simulink model "test_pkt_reord_10_1"  (Simulink 8.0)
settings: Solver=ode45  StartTime=0.0  StopTime=80000  RelTol=1e-3
libraries: xbsIndex_r4 x526, casper_library_misc x11, xps_library x1
(part 1 of 4)
settings Model: Creator=Jason Manley  LastModifiedBy=jmanley
settings DataIOCC: SignalLoggingSaveFormat=ModelDataLogs
settings OptimizationCC: InitFltsAndDblsToZero=on
settings DebuggingCC: FcnCallInpInsideContextMsg=UseLocalSettings  StrictBusMsg=Warning
settings GRTTargetCC: CombineOutputUpdateFcns=off  GRTInterface=on

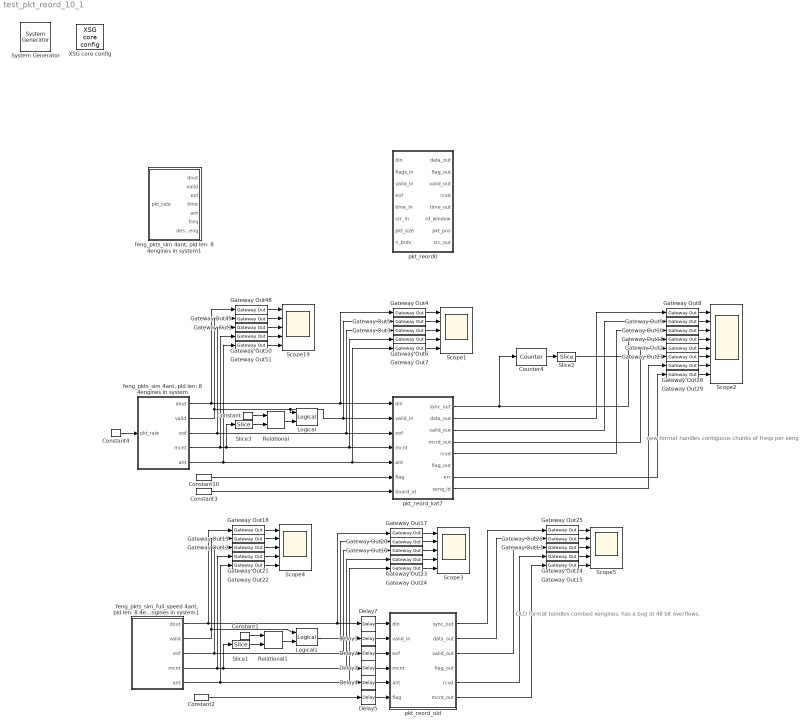
== system test_pkt_reord_10_1 ==
  note: OLD format handles combed
      | xengines. has a bug at 48 bit overflows.
  note: new format handles
      | contiguous chunks of freqs per xeng
  " System Generator" : xbsIndex_r4/ System Generator  Tag=genX  xilinxfamily=virtex2p  part=xc2vp70  speed=-7  package=ff1704  synthesis_tool=XST  clock_wrapper=Clock Enables  directory=./test_pkt_reord_10_1/sysgen  proj_type=Project Navigator  Synth_file=XST Defaults  Impl_file=ISE Defaults  testbench=off  simulink_period=1  sysclk_period=10  dcm_input_clock_period=100  incr_netlist=off  trim_vbits=Everywhere in SubSystem  dbl_ovrd=According to Block Masks  core_generation=According to Block Masks  run_coregen=off  deprecated_control=off  eval_field=0  block_type=sysgen
      settings: block_version=10.1.3
  Constant : xbsIndex_r4/Constant  const=1  gui_display_data_type=Fixed-point  arith_type=Unsigned  n_bits=2  bin_pt=0  preci_type=Single  exp_width=8  frac_width=24  explicit_period=on  period=1  equ=P=C  opselect=C  inp2=PCIN>>17  opr=+  inp1=P  carry=CIN  dbl_ovrd=off  block_type=constant
  Constant1 : xbsIndex_r4/Constant  const=0  gui_display_data_type=Fixed-point  arith_type=Unsigned  n_bits=2  bin_pt=0  preci_type=Single  exp_width=8  frac_width=24  explicit_period=off  period=1  equ=P=C  opselect=C  inp2=PCIN>>17  opr=+  inp1=P  carry=CIN  dbl_ovrd=off  block_type=constant
  Constant10 : xbsIndex_r4/Constant  const=0  gui_display_data_type=Fixed-point  arith_type=Unsigned  n_bits=1  bin_pt=0  preci_type=Single  exp_width=8  frac_width=24  explicit_period=on  period=1  equ=P=C  opselect=C  inp2=PCIN>>17  opr=+  inp1=P  carry=CIN  dbl_ovrd=off  block_type=constant
  Constant2 : xbsIndex_r4/Constant  const=0  gui_display_data_type=Fixed-point  arith_type=Unsigned  n_bits=1  bin_pt=0  preci_type=Single  exp_width=8  frac_width=24  explicit_period=on  period=1  equ=P=C  opselect=C  inp2=PCIN>>17  opr=+  inp1=P  carry=CIN  dbl_ovrd=off  block_type=constant
  Constant3 : xbsIndex_r4/Constant  const=0  gui_display_data_type=Fixed-point  arith_type=Unsigned  n_bits=32  bin_pt=0  preci_type=Single  exp_width=8  frac_width=24  explicit_period=on  period=1  equ=P=C  opselect=C  inp2=PCIN>>17  opr=+  inp1=P  carry=CIN  dbl_ovrd=off  block_type=constant
  Constant4 : xbsIndex_r4/Constant  const=1  gui_display_data_type=Fixed-point  arith_type=Unsigned  n_bits=2  bin_pt=0  preci_type=Single  exp_width=8  frac_width=24  explicit_period=off  period=1  equ=P=C  opselect=C  inp2=PCIN>>17  opr=+  inp1=P  carry=CIN  dbl_ovrd=off  block_type=constant
  Counter4 : xbsIndex_r4/Counter  cnt_type=Free Running  cnt_to=32  operation=Up  start_count=0  cnt_by_val=1  arith_type=Unsigned  n_bits=32  bin_pt=0  load_pin=off  rst=on  en=off  explicit_period=off  period=1  dbl_ovrd=off  use_behavioral_HDL=off  implementation=Fabric  use_rpm=on  block_type=counter
      settings: xl_area=[0, 0, 0, 0, 0, 0, 0]
  Delay{1..5,7} (6 alike) : xbsIndex_r4/Delay  rst=off  infoeditControl=Selection of Reset will increase slice count due to use of real FFs and instead of SRLs  en=off  latency=10  dbl_ovrd=off  reg_retiming=on  block_type=delay
      settings: xl_area=[0, 0, 0, 0, 0, 0, 0]
  Gateway Out{1..29,48..51} (33 alike) : xbsIndex_r4/Gateway Out  inherit_from_input=off  hdl_port=on  timing_constraint=None  locs_specified=off  LOCs={}  UseAsDAC=off  DACChannel='1'  block_type=gatewayout
      settings: infoedit="Gateway out block.  Converts Xilinx fixed point inputs into ouputs of type Simulink integer, double, or fixed point.<P><P>Hardware notes:  In hardware these blocks become top level output ports or are discarded, depending on how they are configured."  xl_area=[0, 0, 0, 0, 0, 0, 0]  block_version=10.1.3
  Logical : xbsIndex_r4/Logical  logical_function=AND  inputs=2  en=off  latency=0  precision=Full  arith_type=Unsigned  n_bits=16  bin_pt=0  align_bp=on  dbl_ovrd=off  block_type=logical
  Logical1 : xbsIndex_r4/Logical  logical_function=AND  inputs=2  en=off  latency=0  precision=Full  arith_type=Unsigned  n_bits=16  bin_pt=0  align_bp=on  dbl_ovrd=off  block_type=logical
  Relational : xbsIndex_r4/Relational  mode=a=b  en=off  latency=1  dbl_ovrd=off  block_type=relational
      settings: block_version=10.1.3
  Relational1 : xbsIndex_r4/Relational  mode=a=b  en=off  latency=1  dbl_ovrd=off  block_type=relational
      settings: block_version=10.1.3
  Scope{1,3..5,19} (5 alike) : Scope  NumInputPorts=5
      Scope1 settings: YMin=2e+14~0~0~0~0  YMax=1.2e+15~1~1~500~3  SaveName=ScopeData6
      Scope19 settings: YMin=0~0~0~0~0  YMax=3e+014~1~1~3000~3  SaveName=ScopeData3
      Scope3 settings: YMin=0~0~0~0~0  YMax=3e+014~1~1~3000~3  SaveName=ScopeData7
      Scope4 settings: YMin=0~0~0~0~0  YMax=3e+014~1~1~3000~3  SaveName=ScopeData8
      Scope5 settings: YMin=0~0~0~-1~-5  YMax=1~1~1~1~5  SaveName=ScopeData9
  Scope2 : Scope  NumInputPorts=8
      settings: YMin=0~0~0~-1~1~30~-1~0  YMax=4~1~1~1~7~90~1~1
  Slice1 : xbsIndex_r4/Slice  nbits=2  boolean_output=off  mode=Lower Bit Location + Width  bit1=0  base1=MSB of Input  bit0=0  base0=LSB of Input  dbl_ovrd=off  block_type=slice
      settings: infoedit="Extracts a given range of bits from each input sample and presents it at the output.  The output type is ordinarily unsigned with binary point at zero, but can be Boolean when the slice is one bit wide.<P><P>Hardware notes: In hardware this block costs nothing."  block_version=10.1.3
  Slice2 : xbsIndex_r4/Slice  nbits=32-(2+5)  boolean_output=off  mode=Lower Bit Location + Width  bit1=0  base1=MSB of Input  bit0=2+5  base0=LSB of Input  dbl_ovrd=off  block_type=slice
      settings: infoedit="Extracts a given range of bits from each input sample and presents it at the output.  The output type is ordinarily unsigned with binary point at zero, but can be Boolean when the slice is one bit wide.<P><P>Hardware notes: In hardware this block costs nothing."  block_version=10.1.3
  Slice3 : xbsIndex_r4/Slice  nbits=2  boolean_output=off  mode=Lower Bit Location + Width  bit1=8  base1=LSB of Input  bit0=6  base0=LSB of Input  dbl_ovrd=off  block_type=slice
      settings: block_version=10.1.3
  XSG core config : xps_library/XSG core config  Tag=xps:xsg  hw_sys=ROACH:sx95t  clk_src=sys_clk  ROACH_clk_src=sys_clk  ROACH2_clk_src=adc0_clk  clk_rate=100  sample_period=1  synthesis_tool=XST
  "feng_pkts_sim 4ant, pld len: 8 4engines in system" : Subsystem
  "feng_pkts_sim 4ant, pld len: 8 4engines in system1" : Subsystem
  "feng_pkts_sim_full_speed 4ant, pld len: 8 4engines in system1" : Subsystem
  pkt_reord0 : Subsystem  mask{window_bits=3, buf_bits=15}
      mask prompts: window_bits "Number of Windows to Buffer (2^?)"; buf_bits "Buffer size (2^?)"
      mask init:
      | fmtstr = sprintf('Buffer space: 2^%i words', buf_bits);
      | set_param(gcb, 'AttributesFormatString', fmtstr);
      settings: AttributesFormatString=Buffer space: 2^15 words
  pkt_reord_kat7 : Subsystem  mask{ant_bits=2, xeng_bits=3, chan_bits=8, x_int_bits=5, window_bits=3, min_sync_bits=5, share_bits=1, nx=0}
      mask prompts: ant_bits "Maximum Number of Antennas (2^?):"; xeng_bits "Number of Xengines in the system (2^?)"; chan_bits "Number of frequency channels in the system (2^?)"; x_int_bits "X Engine Integration Length (2^?):"; window_bits "Number of Windows to Buffer (2^?):"; min_sync_bits "Minimum sync period (2^n)"; share_bits "Number of Xengines on this link (2^?)"; nx "This is engine number"
      mask init:
      | sync_bits=max([min_sync_bits,chan_bits+x_int_bits+ant_bits-xeng_bits]);
      | %sync_bits=chan_bits+x_int_bits+ant_bits-xeng_bits;
      | fmtstr = sprintf('Xeng %d\nSync period: 2^%d\nPayload Len: %i', nx,sync_bits,2^(x_int_bits - 2));
      | set_param(gcb, 'AttributesFormatString', fmtstr);
      settings: AttributesFormatString=|
      | Xeng 0
      | Sync period: 2^12
      | Payload Len: 8
  pkt_reord_old : Subsystem  mask{ant_bits=2, xeng_bits=2, chan_bits=8, x_int_bits=5, window_bits=3, min_sync_bits=5}
      mask prompts: ant_bits "Maximum Number of Antennas (2^?):"; xeng_bits "Number of Xengines in the system (2^?)"; chan_bits "Number of frequency channels in the system (2^?)"; x_int_bits "X Engine Integration Length (2^?):"; window_bits "Number of Windows to Buffer (2^?):"; min_sync_bits "Minimum sync period (2^n)"
      mask init:
      | %sync_bits=max([min_sync_bits,chan_bits+x_int_bits+ant_bits-xeng_bits]);
      | sync_bits=chan_bits+x_int_bits+ant_bits-xeng_bits;
      | fmtstr = sprintf('Sync period: 2^%d\nPayload Len: %i', sync_bits,2^(x_int_bits - 2));
      | set_param(gcb, 'AttributesFormatString', fmtstr);
      settings: AttributesFormatString=|
      | Sync period: 2^13
      | Payload Len: 8
  wires:
  Gateway Out8/1 -> Scope2/1
  Gateway Out9/1 -> Scope2/2
  Gateway Out10/1 -> Scope2/3
  Gateway Out11/1 -> Scope2/4
  pkt_reord_kat7/2(data_out) -> Gateway Out8/1
  pkt_reord_kat7/3(valid_out) -> Gateway Out9/1
  pkt_reord_kat7/5(rcvd) -> Gateway Out10/1
  pkt_reord_kat7/1(sync_out) -> Gateway Out11/1, Counter4/1
  Gateway Out2/1 -> Scope2/5
  pkt_reord_kat7/4(mcnt_out) -> Gateway Out2/1
  Gateway Out48/1 -> Scope19/1
  Gateway Out49/1 -> Scope19/2
  Gateway Out50/1 -> Scope19/4
  Gateway Out51/1 -> Scope19/5
  Gateway Out1/1 -> Scope19/3
  "feng_pkts_sim 4ant, pld len: 8 4engines in system"/1(dout) -> Gateway Out48/1, Gateway Out4/1, pkt_reord_kat7/1(din)
  "feng_pkts_sim 4ant, pld len: 8 4engines in system"/2(valid) -> Gateway Out49/1, Gateway Out5/1, pkt_reord_kat7/2(valid_in), Logical/1
  "feng_pkts_sim 4ant, pld len: 8 4engines in system"/3(eof) -> Gateway Out1/1, Gateway Out3/1, pkt_reord_kat7/3(eof)
  "feng_pkts_sim 4ant, pld len: 8 4engines in system"/4(mcnt) -> Gateway Out50/1, Slice3/1, Gateway Out6/1, pkt_reord_kat7/4(mcnt)
  "feng_pkts_sim 4ant, pld len: 8 4engines in system"/5(ant) -> Gateway Out51/1, Gateway Out7/1, pkt_reord_kat7/5(ant)
  Constant10/1 -> pkt_reord_kat7/6(flag)
  Slice3/1 -> Relational/2
  Constant/1 -> Relational/1
  Relational/1 -> Logical/2
  Gateway Out4/1 -> Scope1/1
  Gateway Out5/1 -> Scope1/2
  Gateway Out6/1 -> Scope1/4
  Gateway Out7/1 -> Scope1/5
  Gateway Out3/1 -> Scope1/3
  Gateway Out25/1 -> Scope5/1
  Gateway Out26/1 -> Scope5/2
  Gateway Out13/1 -> Scope5/3
  Gateway Out14/1 -> Scope5/4
  pkt_reord_old/1(sync_out) -> Gateway Out25/1
  pkt_reord_old/2(data_out) -> Gateway Out26/1
  pkt_reord_old/5(rcvd) -> Gateway Out14/1
  Gateway Out15/1 -> Scope5/5
  pkt_reord_old/6(mcnt_out) -> Gateway Out15/1
  Gateway Out18/1 -> Scope4/1
  Gateway Out19/1 -> Scope4/2
  Gateway Out21/1 -> Scope4/4
  Gateway Out22/1 -> Scope4/5
  Gateway Out12/1 -> Scope4/3
  "feng_pkts_sim_full_speed 4ant, pld len: 8 4engines in system1"/1(dout) -> Gateway Out18/1, Gateway Out17/1, Delay7/1
  "feng_pkts_sim_full_speed 4ant, pld len: 8 4engines in system1"/2(valid) -> Gateway Out19/1, Logical1/1
  "feng_pkts_sim_full_speed 4ant, pld len: 8 4engines in system1"/3(eof) -> Gateway Out12/1, Gateway Out16/1, Delay2/1
  "feng_pkts_sim_full_speed 4ant, pld len: 8 4engines in system1"/4(mcnt) -> Gateway Out21/1, Slice1/1, Gateway Out23/1, Delay3/1
  "feng_pkts_sim_full_speed 4ant, pld len: 8 4engines in system1"/5(ant) -> Gateway Out22/1, Gateway Out24/1, Delay4/1
  Constant2/1 -> Delay5/1
  Logical1/1 -> Gateway Out20/1, Delay1/1
  Slice1/1 -> Relational1/2
  Constant1/1 -> Relational1/1
  Relational1/1 -> Logical1/2
  Gateway Out17/1 -> Scope3/1
  Gateway Out20/1 -> Scope3/2
  Gateway Out23/1 -> Scope3/4
  Gateway Out24/1 -> Scope3/5
  Gateway Out16/1 -> Scope3/3
  Delay7/1 -> pkt_reord_old/1(din)
  Delay1/1 -> pkt_reord_old/2(valid_in)
  Delay2/1 -> pkt_reord_old/3(eof)
  Delay3/1 -> pkt_reord_old/4(mcnt)
  Delay4/1 -> pkt_reord_old/5(ant)
  Delay5/1 -> pkt_reord_old/6(flag)
  pkt_reord_old/3(valid_out) -> Gateway Out13/1
  Counter4/1 -> Slice2/1
  Slice2/1 -> Gateway Out27/1
  Gateway Out27/1 -> Scope2/6
  Constant4/1 -> "feng_pkts_sim 4ant, pld len: 8 4engines in system"/1(pkt_rate)
  Constant3/1 -> pkt_reord_kat7/7(board_id)
  Gateway Out28/1 -> Scope2/7
  Gateway Out29/1 -> Scope2/8
  pkt_reord_kat7/8(xeng_id) -> Gateway Out28/1
  pkt_reord_kat7/7(err) -> Gateway Out29/1

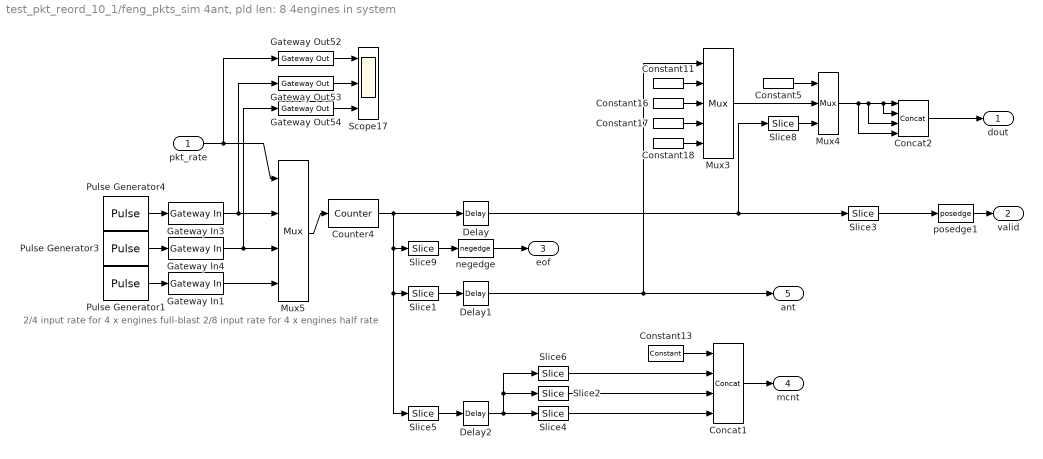
== system test_pkt_reord_10_1/feng_pkts_sim 4ant, pld len: 8 4engines in system ==
  note: 2/4 input rate for 4 x engines full-blast
      | 2/8 input rate for 4 x engines half rate
  pkt_rate : Inport
  Concat1 : xbsIndex_r4/Concat  num_inputs=4  dbl_ovrd=off  block_type=concat
      settings: block_version=10.1.3
  Concat2 : xbsIndex_r4/Concat  num_inputs=4  dbl_ovrd=off  block_type=concat
      settings: block_version=10.1.3
  Constant11 : xbsIndex_r4/Constant  const=1  gui_display_data_type=Fixed-point  arith_type=Unsigned  n_bits=16  bin_pt=0  preci_type=Single  exp_width=8  frac_width=24  explicit_period=on  period=1  equ=P=C  opselect=C  inp2=PCIN>>17  opr=+  inp1=P  carry=CIN  dbl_ovrd=off  block_type=constant
  Constant13 : xbsIndex_r4/Constant  const=0  gui_display_data_type=Fixed-point  arith_type=Unsigned  n_bits=48-(32-6)  bin_pt=0  preci_type=Single  exp_width=8  frac_width=24  explicit_period=on  period=1  equ=P=C  opselect=C  inp2=PCIN>>17  opr=+  inp1=P  carry=CIN  dbl_ovrd=off  block_type=constant
  Constant16 : xbsIndex_r4/Constant  const=2  gui_display_data_type=Fixed-point  arith_type=Unsigned  n_bits=16  bin_pt=0  preci_type=Single  exp_width=8  frac_width=24  explicit_period=on  period=1  equ=P=C  opselect=C  inp2=PCIN>>17  opr=+  inp1=P  carry=CIN  dbl_ovrd=off  block_type=constant
  Constant17 : xbsIndex_r4/Constant  const=3  gui_display_data_type=Fixed-point  arith_type=Unsigned  n_bits=16  bin_pt=0  preci_type=Single  exp_width=8  frac_width=24  explicit_period=on  period=1  equ=P=C  opselect=C  inp2=PCIN>>17  opr=+  inp1=P  carry=CIN  dbl_ovrd=off  block_type=constant
  Constant18 : xbsIndex_r4/Constant  const=4  gui_display_data_type=Fixed-point  arith_type=Unsigned  n_bits=16  bin_pt=0  preci_type=Single  exp_width=8  frac_width=24  explicit_period=on  period=1  equ=P=C  opselect=C  inp2=PCIN>>17  opr=+  inp1=P  carry=CIN  dbl_ovrd=off  block_type=constant
  Constant5 : xbsIndex_r4/Constant  const=0  gui_display_data_type=Fixed-point  arith_type=Unsigned  n_bits=1  bin_pt=0  preci_type=Single  exp_width=8  frac_width=24  explicit_period=on  period=1  equ=P=C  opselect=C  inp2=PCIN>>17  opr=+  inp1=P  carry=CIN  dbl_ovrd=off  block_type=constant
  Counter4 : xbsIndex_r4/Counter  cnt_type=Free Running  cnt_to=32  operation=Up  start_count=0  cnt_by_val=1  arith_type=Unsigned  n_bits=32  bin_pt=0  load_pin=off  rst=off  en=on  explicit_period=off  period=1  dbl_ovrd=off  use_behavioral_HDL=off  implementation=Fabric  use_rpm=on  block_type=counter
      settings: xl_area=[0, 0, 0, 0, 0, 0, 0]
  Delay : xbsIndex_r4/Delay  rst=off  infoeditControl=Selection of Reset will increase slice count due to use of real FFs and instead of SRLs  en=off  latency=1  dbl_ovrd=off  reg_retiming=off  block_type=delay
      settings: xl_area=[0, 0, 0, 0, 0, 0, 0]
  Delay1 : xbsIndex_r4/Delay  rst=off  infoeditControl=Selection of Reset will increase slice count due to use of real FFs and instead of SRLs  en=off  latency=1  dbl_ovrd=off  reg_retiming=off  block_type=delay
      settings: xl_area=[0, 0, 0, 0, 0, 0, 0]
  Delay2 : xbsIndex_r4/Delay  rst=off  infoeditControl=Selection of Reset will increase slice count due to use of real FFs and instead of SRLs  en=off  latency=1  dbl_ovrd=off  reg_retiming=off  block_type=delay
      settings: xl_area=[0, 0, 0, 0, 0, 0, 0]
  Gateway In1 : xbsIndex_r4/Gateway In  gui_display_data_type=Fixed-point  arith_type=Boolean  n_bits=8  bin_pt=6  preci_type=Single  exp_width=8  frac_width=24  quantization=Truncate  overflow=Wrap  period=1  dbl_ovrd=off  timing_constraint=None  locs_specified=off  LOCs={}  UseAsADC=off  ADCChannel='1'  inherit_from_input=off  hdl_port=on  block_type=gatewayin
      settings: infoedit="Gateway in block.  Converts inputs of type Simulink integer, double and fixed point to  Xilinx fixed point type.<P><P>Hardware notes:  In hardware these blocks become top level input ports."  xl_area=[0, 0, 0, 0, 0, 0, 0]  block_version=10.1.3
  Gateway In3 : xbsIndex_r4/Gateway In  gui_display_data_type=Fixed-point  arith_type=Boolean  n_bits=8  bin_pt=6  preci_type=Single  exp_width=8  frac_width=24  quantization=Truncate  overflow=Wrap  period=1  dbl_ovrd=off  timing_constraint=None  locs_specified=off  LOCs={}  UseAsADC=off  ADCChannel='1'  inherit_from_input=off  hdl_port=on  block_type=gatewayin
      settings: infoedit="Gateway in block.  Converts inputs of type Simulink integer, double and fixed point to  Xilinx fixed point type.<P><P>Hardware notes:  In hardware these blocks become top level input ports."  xl_area=[0, 0, 0, 0, 0, 0, 0]  block_version=10.1.3
  Gateway In4 : xbsIndex_r4/Gateway In  gui_display_data_type=Fixed-point  arith_type=Boolean  n_bits=8  bin_pt=6  preci_type=Single  exp_width=8  frac_width=24  quantization=Truncate  overflow=Wrap  period=1  dbl_ovrd=off  timing_constraint=None  locs_specified=off  LOCs={}  UseAsADC=off  ADCChannel='1'  inherit_from_input=off  hdl_port=on  block_type=gatewayin
      settings: infoedit="Gateway in block.  Converts inputs of type Simulink integer, double and fixed point to  Xilinx fixed point type.<P><P>Hardware notes:  In hardware these blocks become top level input ports."  xl_area=[0, 0, 0, 0, 0, 0, 0]  block_version=10.1.3
  Gateway Out52 : xbsIndex_r4/Gateway Out  inherit_from_input=off  hdl_port=on  timing_constraint=None  locs_specified=off  LOCs={}  UseAsDAC=off  DACChannel='1'  block_type=gatewayout
      settings: infoedit="Gateway out block.  Converts Xilinx fixed point inputs into ouputs of type Simulink integer, double, or fixed point.<P><P>Hardware notes:  In hardware these blocks become top level output ports or are discarded, depending on how they are configured."  xl_area=[0, 0, 0, 0, 0, 0, 0]  block_version=10.1.3
  Gateway Out53 : xbsIndex_r4/Gateway Out  inherit_from_input=off  hdl_port=on  timing_constraint=None  locs_specified=off  LOCs={}  UseAsDAC=off  DACChannel='1'  block_type=gatewayout
      settings: infoedit="Gateway out block.  Converts Xilinx fixed point inputs into ouputs of type Simulink integer, double, or fixed point.<P><P>Hardware notes:  In hardware these blocks become top level output ports or are discarded, depending on how they are configured."  xl_area=[0, 0, 0, 0, 0, 0, 0]  block_version=10.1.3
  Gateway Out54 : xbsIndex_r4/Gateway Out  inherit_from_input=off  hdl_port=on  timing_constraint=None  locs_specified=off  LOCs={}  UseAsDAC=off  DACChannel='1'  block_type=gatewayout
      settings: infoedit="Gateway out block.  Converts Xilinx fixed point inputs into ouputs of type Simulink integer, double, or fixed point.<P><P>Hardware notes:  In hardware these blocks become top level output ports or are discarded, depending on how they are configured."  xl_area=[0, 0, 0, 0, 0, 0, 0]  block_version=10.1.3
  Mux3 : xbsIndex_r4/Mux  inputs=4  en=off  latency=0  precision=Full  arith_type="Signed  (2's comp)"  n_bits=8  bin_pt=2  quantization=Truncate  overflow=Wrap  dbl_ovrd=off  block_type=mux
      settings: xl_area=[0, 0, 0, 0, 0, 0, 0]
  Mux4 : xbsIndex_r4/Mux  inputs=2  en=off  latency=0  precision=Full  arith_type="Signed  (2's comp)"  n_bits=8  bin_pt=2  quantization=Truncate  overflow=Wrap  dbl_ovrd=off  block_type=mux
      settings: xl_area=[0, 0, 0, 0, 0, 0, 0]
  Mux5 : xbsIndex_r4/Mux  inputs=3  en=off  latency=0  precision=Full  arith_type="Signed  (2's comp)"  n_bits=8  bin_pt=2  quantization=Truncate  overflow=Wrap  dbl_ovrd=off  block_type=mux
      settings: xl_area=[0, 0, 0, 0, 0, 0, 0]
  Pulse Generator1 : DiscretePulseGenerator  PulseWidth=2
  Pulse Generator3 : DiscretePulseGenerator  Period=4  PulseWidth=2
  Pulse Generator4 : DiscretePulseGenerator  Period=8  PulseWidth=2
  Scope17 : Scope  NumInputPorts=3
      settings: YMin=-1~0~0  YMax=1~1~1
  Slice1 : xbsIndex_r4/Slice  nbits=2  boolean_output=off  mode=Lower Bit Location + Width  bit1=0  base1=MSB of Input  bit0=4  base0=LSB of Input  dbl_ovrd=off  block_type=slice
      settings: infoedit="Extracts a given range of bits from each input sample and presents it at the output.  The output type is ordinarily unsigned with binary point at zero, but can be Boolean when the slice is one bit wide.<P><P>Hardware notes: In hardware this block costs nothing."  block_version=10.1.3
  Slice2 : xbsIndex_r4/Slice  nbits=3  boolean_output=off  mode=Lower Bit Location + Width  bit1=4+2+2  base1=LSB of Input  bit0=0  base0=LSB of Input  dbl_ovrd=off  block_type=slice
      settings: block_version=10.1.3
  Slice3 : xbsIndex_r4/Slice  nbits=1  boolean_output=on  mode=Lower Bit Location + Width  bit1=0  base1=MSB of Input  bit0=0  base0=LSB of Input  dbl_ovrd=off  block_type=slice
      settings: infoedit="Extracts a given range of bits from each input sample and presents it at the output.  The output type is ordinarily unsigned with binary point at zero, but can be Boolean when the slice is one bit wide.<P><P>Hardware notes: In hardware this block costs nothing."  block_version=10.1.3
  Slice4 : xbsIndex_r4/Slice  nbits=5  boolean_output=off  mode=Lower Bit Location + Width  bit1=0  base1=MSB of Input  bit0=3  base0=LSB of Input  dbl_ovrd=off  block_type=slice
      settings: block_version=10.1.3
  Slice5 : xbsIndex_r4/Slice  nbits=48  boolean_output=off  mode=Two Bit Locations  bit1=0  base1=MSB of Input  bit0=6  base0=LSB of Input  dbl_ovrd=off  block_type=slice
      settings: block_version=10.1.3
  Slice6 : xbsIndex_r4/Slice  nbits=10  boolean_output=off  mode=Two Bit Locations  bit1=0  base1=MSB of Input  bit0=8  base0=LSB of Input  dbl_ovrd=off  block_type=slice
      settings: block_version=10.1.3
  Slice8 : xbsIndex_r4/Slice  nbits=16  boolean_output=off  mode=Lower Bit Location + Width  bit1=0  base1=MSB of Input  bit0=1  base0=LSB of Input  dbl_ovrd=off  block_type=slice
      settings: infoedit="Extracts a given range of bits from each input sample and presents it at the output.  The output type is ordinarily unsigned with binary point at zero, but can be Boolean when the slice is one bit wide.<P><P>Hardware notes: In hardware this block costs nothing."  block_version=10.1.3
  Slice9 : xbsIndex_r4/Slice  nbits=1  boolean_output=on  mode=Lower Bit Location + Width  bit1=0  base1=MSB of Input  bit0=3  base0=LSB of Input  dbl_ovrd=off  block_type=slice
      settings: infoedit="Extracts a given range of bits from each input sample and presents it at the output.  The output type is ordinarily unsigned with binary point at zero, but can be Boolean when the slice is one bit wide.<P><P>Hardware notes: In hardware this block costs nothing."  block_version=10.1.3
  negedge : casper_library_misc/negedge  Tag=Rising Edge Detector
  posedge1 : casper_library_misc/posedge  Tag=Rising Edge Detector
  dout : Outport
  valid : Outport  Port=2
  eof : Outport  Port=3
  mcnt : Outport  Port=4
  ant : Outport  Port=5
  wires:
  Delay/1 -> Slice8/1, Slice3/1
  Concat1/1 -> mcnt/1
  posedge1/1 -> valid/1
  Concat2/1 -> dout/1
  Gateway Out54/1 -> Scope17/3
  Gateway Out53/1 -> Scope17/2
  Gateway Out52/1 -> Scope17/1
  pkt_rate/1 -> Mux5/1, Gateway Out52/1
  Gateway In4/1 -> Mux5/3, Gateway Out54/1
  Gateway In3/1 -> Mux5/2, Gateway Out53/1
  Mux5/1 -> Counter4/1
  Pulse Generator4/1 -> Gateway In3/1
  Constant5/1 -> Mux4/1
  Slice8/1 -> Mux4/3
  Mux3/1 -> Mux4/2
  Constant18/1 -> Mux3/5
  Constant17/1 -> Mux3/4
  Constant16/1 -> Mux3/3
  Constant11/1 -> Mux3/2
  Pulse Generator3/1 -> Gateway In4/1
  negedge/1 -> eof/1
  Slice9/1 -> negedge/1
  Mux4/1 -> Concat2/2, Concat2/1, Concat2/3, Concat2/4
  Counter4/1 -> Delay/1, Slice9/1, Slice1/1, Slice5/1
  Slice3/1 -> posedge1/1
  Slice1/1 -> Delay1/1
  Delay1/1 -> ant/1, Mux3/1
  Constant13/1 -> Concat1/1
  Pulse Generator1/1 -> Gateway In1/1
  Gateway In1/1 -> Mux5/4
  Delay2/1 -> Slice4/1, Slice2/1, Slice6/1
  Slice5/1 -> Delay2/1
  Slice6/1 -> Concat1/2
  Slice2/1 -> Concat1/3
  Slice4/1 -> Concat1/4

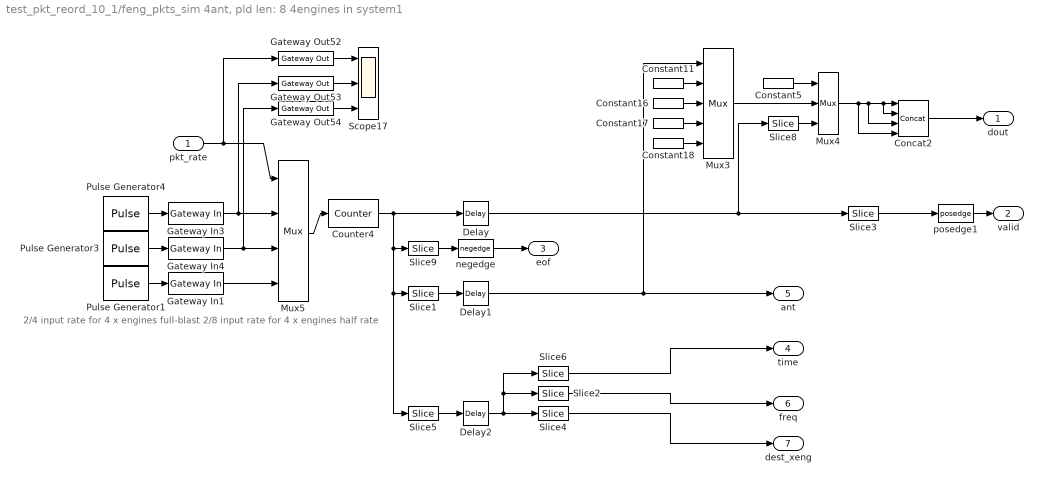
== system test_pkt_reord_10_1/feng_pkts_sim 4ant, pld len: 8 4engines in system1 ==
  note: 2/4 input rate for 4 x engines full-blast
      | 2/8 input rate for 4 x engines half rate
  pkt_rate : Inport
  Concat2 : xbsIndex_r4/Concat  num_inputs=4  dbl_ovrd=off  block_type=concat
      settings: block_version=10.1.3
  Constant11 : xbsIndex_r4/Constant  const=1  gui_display_data_type=Fixed-point  arith_type=Unsigned  n_bits=16  bin_pt=0  preci_type=Single  exp_width=8  frac_width=24  explicit_period=on  period=1  equ=P=C  opselect=C  inp2=PCIN>>17  opr=+  inp1=P  carry=CIN  dbl_ovrd=off  block_type=constant
  Constant16 : xbsIndex_r4/Constant  const=2  gui_display_data_type=Fixed-point  arith_type=Unsigned  n_bits=16  bin_pt=0  preci_type=Single  exp_width=8  frac_width=24  explicit_period=on  period=1  equ=P=C  opselect=C  inp2=PCIN>>17  opr=+  inp1=P  carry=CIN  dbl_ovrd=off  block_type=constant
  Constant17 : xbsIndex_r4/Constant  const=3  gui_display_data_type=Fixed-point  arith_type=Unsigned  n_bits=16  bin_pt=0  preci_type=Single  exp_width=8  frac_width=24  explicit_period=on  period=1  equ=P=C  opselect=C  inp2=PCIN>>17  opr=+  inp1=P  carry=CIN  dbl_ovrd=off  block_type=constant
  Constant18 : xbsIndex_r4/Constant  const=4  gui_display_data_type=Fixed-point  arith_type=Unsigned  n_bits=16  bin_pt=0  preci_type=Single  exp_width=8  frac_width=24  explicit_period=on  period=1  equ=P=C  opselect=C  inp2=PCIN>>17  opr=+  inp1=P  carry=CIN  dbl_ovrd=off  block_type=constant
  Constant5 : xbsIndex_r4/Constant  const=0  gui_display_data_type=Fixed-point  arith_type=Unsigned  n_bits=1  bin_pt=0  preci_type=Single  exp_width=8  frac_width=24  explicit_period=on  period=1  equ=P=C  opselect=C  inp2=PCIN>>17  opr=+  inp1=P  carry=CIN  dbl_ovrd=off  block_type=constant
  Counter4 : xbsIndex_r4/Counter  cnt_type=Free Running  cnt_to=32  operation=Up  start_count=0  cnt_by_val=1  arith_type=Unsigned  n_bits=32  bin_pt=0  load_pin=off  rst=off  en=on  explicit_period=off  period=1  dbl_ovrd=off  use_behavioral_HDL=off  implementation=Fabric  use_rpm=on  block_type=counter
      settings: xl_area=[0, 0, 0, 0, 0, 0, 0]
  Delay : xbsIndex_r4/Delay  rst=off  infoeditControl=Selection of Reset will increase slice count due to use of real FFs and instead of SRLs  en=off  latency=1  dbl_ovrd=off  reg_retiming=off  block_type=delay
      settings: xl_area=[0, 0, 0, 0, 0, 0, 0]
  Delay1 : xbsIndex_r4/Delay  rst=off  infoeditControl=Selection of Reset will increase slice count due to use of real FFs and instead of SRLs  en=off  latency=1  dbl_ovrd=off  reg_retiming=off  block_type=delay
      settings: xl_area=[0, 0, 0, 0, 0, 0, 0]
  Delay2 : xbsIndex_r4/Delay  rst=off  infoeditControl=Selection of Reset will increase slice count due to use of real FFs and instead of SRLs  en=off  latency=1  dbl_ovrd=off  reg_retiming=off  block_type=delay
      settings: xl_area=[0, 0, 0, 0, 0, 0, 0]
  Gateway In1 : xbsIndex_r4/Gateway In  gui_display_data_type=Fixed-point  arith_type=Boolean  n_bits=8  bin_pt=6  preci_type=Single  exp_width=8  frac_width=24  quantization=Truncate  overflow=Wrap  period=1  dbl_ovrd=off  timing_constraint=None  locs_specified=off  LOCs={}  UseAsADC=off  ADCChannel='1'  inherit_from_input=off  hdl_port=on  block_type=gatewayin
      settings: infoedit="Gateway in block.  Converts inputs of type Simulink integer, double and fixed point to  Xilinx fixed point type.<P><P>Hardware notes:  In hardware these blocks become top level input ports."  xl_area=[0, 0, 0, 0, 0, 0, 0]  block_version=10.1.3
  Gateway In3 : xbsIndex_r4/Gateway In  gui_display_data_type=Fixed-point  arith_type=Boolean  n_bits=8  bin_pt=6  preci_type=Single  exp_width=8  frac_width=24  quantization=Truncate  overflow=Wrap  period=1  dbl_ovrd=off  timing_constraint=None  locs_specified=off  LOCs={}  UseAsADC=off  ADCChannel='1'  inherit_from_input=off  hdl_port=on  block_type=gatewayin
      settings: infoedit="Gateway in block.  Converts inputs of type Simulink integer, double and fixed point to  Xilinx fixed point type.<P><P>Hardware notes:  In hardware these blocks become top level input ports."  xl_area=[0, 0, 0, 0, 0, 0, 0]  block_version=10.1.3
  Gateway In4 : xbsIndex_r4/Gateway In  gui_display_data_type=Fixed-point  arith_type=Boolean  n_bits=8  bin_pt=6  preci_type=Single  exp_width=8  frac_width=24  quantization=Truncate  overflow=Wrap  period=1  dbl_ovrd=off  timing_constraint=None  locs_specified=off  LOCs={}  UseAsADC=off  ADCChannel='1'  inherit_from_input=off  hdl_port=on  block_type=gatewayin
      settings: infoedit="Gateway in block.  Converts inputs of type Simulink integer, double and fixed point to  Xilinx fixed point type.<P><P>Hardware notes:  In hardware these blocks become top level input ports."  xl_area=[0, 0, 0, 0, 0, 0, 0]  block_version=10.1.3
  Gateway Out52 : xbsIndex_r4/Gateway Out  inherit_from_input=off  hdl_port=on  timing_constraint=None  locs_specified=off  LOCs={}  UseAsDAC=off  DACChannel='1'  block_type=gatewayout
      settings: infoedit="Gateway out block.  Converts Xilinx fixed point inputs into ouputs of type Simulink integer, double, or fixed point.<P><P>Hardware notes:  In hardware these blocks become top level output ports or are discarded, depending on how they are configured."  xl_area=[0, 0, 0, 0, 0, 0, 0]  block_version=10.1.3
  Gateway Out53 : xbsIndex_r4/Gateway Out  inherit_from_input=off  hdl_port=on  timing_constraint=None  locs_specified=off  LOCs={}  UseAsDAC=off  DACChannel='1'  block_type=gatewayout
      settings: infoedit="Gateway out block.  Converts Xilinx fixed point inputs into ouputs of type Simulink integer, double, or fixed point.<P><P>Hardware notes:  In hardware these blocks become top level output ports or are discarded, depending on how they are configured."  xl_area=[0, 0, 0, 0, 0, 0, 0]  block_version=10.1.3
  Gateway Out54 : xbsIndex_r4/Gateway Out  inherit_from_input=off  hdl_port=on  timing_constraint=None  locs_specified=off  LOCs={}  UseAsDAC=off  DACChannel='1'  block_type=gatewayout
      settings: infoedit="Gateway out block.  Converts Xilinx fixed point inputs into ouputs of type Simulink integer, double, or fixed point.<P><P>Hardware notes:  In hardware these blocks become top level output ports or are discarded, depending on how they are configured."  xl_area=[0, 0, 0, 0, 0, 0, 0]  block_version=10.1.3
  Mux3 : xbsIndex_r4/Mux  inputs=4  en=off  latency=0  precision=Full  arith_type="Signed  (2's comp)"  n_bits=8  bin_pt=2  quantization=Truncate  overflow=Wrap  dbl_ovrd=off  block_type=mux
      settings: xl_area=[0, 0, 0, 0, 0, 0, 0]
  Mux4 : xbsIndex_r4/Mux  inputs=2  en=off  latency=0  precision=Full  arith_type="Signed  (2's comp)"  n_bits=8  bin_pt=2  quantization=Truncate  overflow=Wrap  dbl_ovrd=off  block_type=mux
      settings: xl_area=[0, 0, 0, 0, 0, 0, 0]
  Mux5 : xbsIndex_r4/Mux  inputs=3  en=off  latency=0  precision=Full  arith_type="Signed  (2's comp)"  n_bits=8  bin_pt=2  quantization=Truncate  overflow=Wrap  dbl_ovrd=off  block_type=mux
      settings: xl_area=[0, 0, 0, 0, 0, 0, 0]
  Pulse Generator1 : DiscretePulseGenerator  PulseWidth=2
  Pulse Generator3 : DiscretePulseGenerator  Period=4  PulseWidth=2
  Pulse Generator4 : DiscretePulseGenerator  Period=8  PulseWidth=2
  Scope17 : Scope  NumInputPorts=3
      settings: YMin=-1~0~0  YMax=1~1~1
  Slice1 : xbsIndex_r4/Slice  nbits=2  boolean_output=off  mode=Lower Bit Location + Width  bit1=0  base1=MSB of Input  bit0=4  base0=LSB of Input  dbl_ovrd=off  block_type=slice
      settings: infoedit="Extracts a given range of bits from each input sample and presents it at the output.  The output type is ordinarily unsigned with binary point at zero, but can be Boolean when the slice is one bit wide.<P><P>Hardware notes: In hardware this block costs nothing."  block_version=10.1.3
  Slice2 : xbsIndex_r4/Slice  nbits=3  boolean_output=off  mode=Lower Bit Location + Width  bit1=4+2+2  base1=LSB of Input  bit0=0  base0=LSB of Input  dbl_ovrd=off  block_type=slice
      settings: block_version=10.1.3
  Slice3 : xbsIndex_r4/Slice  nbits=1  boolean_output=on  mode=Lower Bit Location + Width  bit1=0  base1=MSB of Input  bit0=0  base0=LSB of Input  dbl_ovrd=off  block_type=slice
      settings: infoedit="Extracts a given range of bits from each input sample and presents it at the output.  The output type is ordinarily unsigned with binary point at zero, but can be Boolean when the slice is one bit wide.<P><P>Hardware notes: In hardware this block costs nothing."  block_version=10.1.3
  Slice4 : xbsIndex_r4/Slice  nbits=5  boolean_output=off  mode=Lower Bit Location + Width  bit1=0  base1=MSB of Input  bit0=3  base0=LSB of Input  dbl_ovrd=off  block_type=slice
      settings: block_version=10.1.3
  Slice5 : xbsIndex_r4/Slice  nbits=48  boolean_output=off  mode=Two Bit Locations  bit1=0  base1=MSB of Input  bit0=6  base0=LSB of Input  dbl_ovrd=off  block_type=slice
      settings: block_version=10.1.3
  Slice6 : xbsIndex_r4/Slice  nbits=10  boolean_output=off  mode=Two Bit Locations  bit1=0  base1=MSB of Input  bit0=8  base0=LSB of Input  dbl_ovrd=off  block_type=slice
      settings: block_version=10.1.3
  Slice8 : xbsIndex_r4/Slice  nbits=16  boolean_output=off  mode=Lower Bit Location + Width  bit1=0  base1=MSB of Input  bit0=1  base0=LSB of Input  dbl_ovrd=off  block_type=slice
      settings: infoedit="Extracts a given range of bits from each input sample and presents it at the output.  The output type is ordinarily unsigned with binary point at zero, but can be Boolean when the slice is one bit wide.<P><P>Hardware notes: In hardware this block costs nothing."  block_version=10.1.3
  Slice9 : xbsIndex_r4/Slice  nbits=1  boolean_output=on  mode=Lower Bit Location + Width  bit1=0  base1=MSB of Input  bit0=3  base0=LSB of Input  dbl_ovrd=off  block_type=slice
      settings: infoedit="Extracts a given range of bits from each input sample and presents it at the output.  The output type is ordinarily unsigned with binary point at zero, but can be Boolean when the slice is one bit wide.<P><P>Hardware notes: In hardware this block costs nothing."  block_version=10.1.3
  negedge : casper_library_misc/negedge  Tag=Rising Edge Detector
  posedge1 : casper_library_misc/posedge  Tag=Rising Edge Detector
  dout : Outport
  valid : Outport  Port=2
  eof : Outport  Port=3
  time : Outport  Port=4
  ant : Outport  Port=5
  freq : Outport  Port=6
  dest_xeng : Outport  Port=7
  wires:
  Slice5/1 -> Delay2/1
  Delay2/1 -> Slice6/1, Slice2/1, Slice4/1
  Gateway In1/1 -> Mux5/4
  Pulse Generator1/1 -> Gateway In1/1
  Delay1/1 -> Mux3/1, ant/1
  Slice1/1 -> Delay1/1
  Slice3/1 -> posedge1/1
  Counter4/1 -> Slice5/1, Slice1/1, Slice9/1, Delay/1
  Mux4/1 -> Concat2/4, Concat2/3, Concat2/1, Concat2/2
  Slice9/1 -> negedge/1
  negedge/1 -> eof/1
  Pulse Generator3/1 -> Gateway In4/1
  Constant11/1 -> Mux3/2
  Constant16/1 -> Mux3/3
  Constant17/1 -> Mux3/4
  Constant18/1 -> Mux3/5
  Mux3/1 -> Mux4/2
  Slice8/1 -> Mux4/3
  Constant5/1 -> Mux4/1
  Pulse Generator4/1 -> Gateway In3/1
  Mux5/1 -> Counter4/1
  Gateway In3/1 -> Gateway Out53/1, Mux5/2
  Gateway In4/1 -> Gateway Out54/1, Mux5/3
  pkt_rate/1 -> Gateway Out52/1, Mux5/1
  Gateway Out52/1 -> Scope17/1
  Gateway Out53/1 -> Scope17/2
  Gateway Out54/1 -> Scope17/3
  Concat2/1 -> dout/1
  posedge1/1 -> valid/1
  Delay/1 -> Slice3/1, Slice8/1
  Slice2/1 -> freq/1
  Slice6/1 -> time/1
  Slice4/1 -> dest_xeng/1

== system test_pkt_reord_10_1/feng_pkts_sim_full_speed 4ant, pld len: 8 4engines in system1 ==
  Concat1 : xbsIndex_r4/Concat  num_inputs=2  dbl_ovrd=off  block_type=concat
      settings: block_version=10.1.3
  Concat2 : xbsIndex_r4/Concat  num_inputs=4  dbl_ovrd=off  block_type=concat
      settings: block_version=10.1.3
  Constant1 : xbsIndex_r4/Constant  arith_type=Boolean  const=1  n_bits=48-(32-6)  bin_pt=0  explicit_period=on  period=1  equ=P=C  opselect=C  inp2=PCIN>>17  opr=+  inp1=P  carry=CIN  dbl_ovrd=off  block_type=constant
  Constant11 : xbsIndex_r4/Constant  arith_type=Unsigned  const=1  n_bits=16  bin_pt=0  explicit_period=on  period=1  equ=P=C  opselect=C  inp2=PCIN>>17  opr=+  inp1=P  carry=CIN  dbl_ovrd=off  block_type=constant
  Constant13 : xbsIndex_r4/Constant  arith_type=Unsigned  const=0  n_bits=48-(32-5)  bin_pt=0  explicit_period=on  period=1  equ=P=C  opselect=C  inp2=PCIN>>17  opr=+  inp1=P  carry=CIN  dbl_ovrd=off  block_type=constant
  Constant16 : xbsIndex_r4/Constant  arith_type=Unsigned  const=0  n_bits=16  bin_pt=0  explicit_period=on  period=1  equ=P=C  opselect=C  inp2=PCIN>>17  opr=+  inp1=P  carry=CIN  dbl_ovrd=off  block_type=constant
  Constant17 : xbsIndex_r4/Constant  arith_type=Unsigned  const=0  n_bits=16  bin_pt=0  explicit_period=on  period=1  equ=P=C  opselect=C  inp2=PCIN>>17  opr=+  inp1=P  carry=CIN  dbl_ovrd=off  block_type=constant
  Constant18 : xbsIndex_r4/Constant  arith_type=Unsigned  const=0  n_bits=16  bin_pt=0  explicit_period=on  period=1  equ=P=C  opselect=C  inp2=PCIN>>17  opr=+  inp1=P  carry=CIN  dbl_ovrd=off  block_type=constant
  Constant5 : xbsIndex_r4/Constant  arith_type=Unsigned  const=0  n_bits=1  bin_pt=0  explicit_period=on  period=1  equ=P=C  opselect=C  inp2=PCIN>>17  opr=+  inp1=P  carry=CIN  dbl_ovrd=off  block_type=constant
  Counter4 : xbsIndex_r4/Counter  cnt_type=Free Running  cnt_to=32  operation=Up  start_count=0  cnt_by_val=1  arith_type=Unsigned  n_bits=32  bin_pt=0  load_pin=off  rst=off  en=off  explicit_period=on  period=1  dbl_ovrd=off  use_behavioral_HDL=off  implementation=Fabric  use_rpm=on  block_type=counter
      settings: xl_area=[0, 0, 0, 0, 0, 0, 0]
  Delay : xbsIndex_r4/Delay  en=off  latency=1  dbl_ovrd=off  reg_retiming=off  block_type=delay
      settings: xl_area=[0, 0, 0, 0, 0, 0, 0]
  Delay1 : xbsIndex_r4/Delay  en=off  latency=1  dbl_ovrd=off  reg_retiming=off  block_type=delay
      settings: xl_area=[0, 0, 0, 0, 0, 0, 0]
  Delay2 : xbsIndex_r4/Delay  en=off  latency=1  dbl_ovrd=off  reg_retiming=off  block_type=delay
      settings: xl_area=[0, 0, 0, 0, 0, 0, 0]
  Mux3 : xbsIndex_r4/Mux  inputs=4  en=off  latency=0  precision=Full  arith_type="Signed  (2's comp)"  n_bits=8  bin_pt=2  quantization=Truncate  overflow=Wrap  dbl_ovrd=off  block_type=mux
      settings: xl_area=[0, 0, 0, 0, 0, 0, 0]
  Mux4 : xbsIndex_r4/Mux  inputs=2  en=off  latency=0  precision=Full  arith_type="Signed  (2's comp)"  n_bits=8  bin_pt=2  quantization=Truncate  overflow=Wrap  dbl_ovrd=off  block_type=mux
      settings: xl_area=[0, 0, 0, 0, 0, 0, 0]
  Slice1 : xbsIndex_r4/Slice  nbits=2  boolean_output=off  mode=Lower Bit Location + Width  bit1=0  base1=MSB of Input  bit0=3  base0=LSB of Input  dbl_ovrd=off  block_type=slice
      settings: infoedit="Extracts a given range of bits from each input sample and presents it at the output.  The output type is ordinarily unsigned with binary point at zero, but can be Boolean when the slice is one bit wide.<P><P>Hardware notes: In hardware this block costs nothing."  block_version=10.1.3
  Slice2 : xbsIndex_r4/Slice  nbits=48  boolean_output=off  mode=Two Bit Locations  bit1=0  base1=MSB of Input  bit0=4+1  base0=LSB of Input  dbl_ovrd=off  block_type=slice
      settings: infoedit="Extracts a given range of bits from each input sample and presents it at the output.  The output type is ordinarily unsigned with binary point at zero, but can be Boolean when the slice is one bit wide.<P><P>Hardware notes: In hardware this block costs nothing."  block_version=10.1.3
  Slice8 : xbsIndex_r4/Slice  nbits=16  boolean_output=off  mode=Lower Bit Location + Width  bit1=0  base1=MSB of Input  bit0=1  base0=LSB of Input  dbl_ovrd=off  block_type=slice
      settings: infoedit="Extracts a given range of bits from each input sample and presents it at the output.  The output type is ordinarily unsigned with binary point at zero, but can be Boolean when the slice is one bit wide.<P><P>Hardware notes: In hardware this block costs nothing."  block_version=10.1.3
  Slice9 : xbsIndex_r4/Slice  nbits=1  boolean_output=on  mode=Lower Bit Location + Width  bit1=0  base1=MSB of Input  bit0=2  base0=LSB of Input  dbl_ovrd=off  block_type=slice
      settings: infoedit="Extracts a given range of bits from each input sample and presents it at the output.  The output type is ordinarily unsigned with binary point at zero, but can be Boolean when the slice is one bit wide.<P><P>Hardware notes: In hardware this block costs nothing."  block_version=10.1.3
  negedge : casper_library_misc/negedge  Tag=Rising Edge Detector  SystemSampleTime=-1
  dout : Outport
  valid : Outport  Port=2
  eof : Outport  Port=3
  mcnt : Outport  Port=4
  ant : Outport  Port=5
  wires:
  Delay2/1 -> Concat1/2
  Constant13/1 -> Concat1/1
  Delay1/1 -> Mux3/1, ant/1
  Slice2/1 -> Delay2/1
  Slice1/1 -> Delay1/1
  Counter4/1 -> Slice2/1, Slice1/1, Slice9/1, Delay/1
  Mux4/1 -> Concat2/4, Concat2/3, Concat2/1, Concat2/2
  Slice9/1 -> negedge/1
  negedge/1 -> eof/1
  Constant11/1 -> Mux3/2
  Constant16/1 -> Mux3/3
  Constant17/1 -> Mux3/4
  Constant18/1 -> Mux3/5
  Mux3/1 -> Mux4/2
  Slice8/1 -> Mux4/3
  Constant5/1 -> Mux4/1
  Concat2/1 -> dout/1
  Concat1/1 -> mcnt/1
  Delay/1 -> Slice8/1
  Constant1/1 -> valid/1

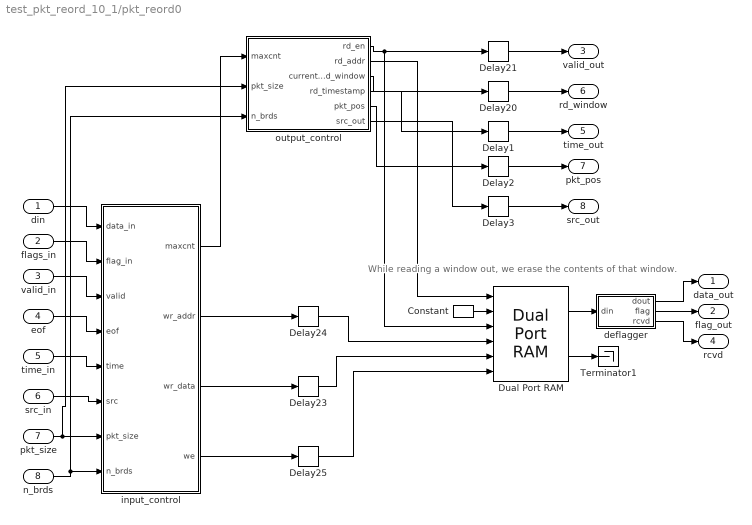
== system test_pkt_reord_10_1/pkt_reord0 ==
  note: While reading a window out,
      | we erase the contents of that window.
  din : Inport
  flags_in : Inport  Port=2
  valid_in : Inport  Port=3
  eof : Inport  Port=4
  time_in : Inport  Port=5
  src_in : Inport  Port=6
  pkt_size : Inport  Port=7
  n_brds : Inport  Port=8
  Constant : xbsIndex_r4/Constant  const=0  gui_display_data_type=Fixed-point  arith_type=Unsigned  n_bits=72  bin_pt=0  preci_type=Single  exp_width=8  frac_width=24  explicit_period=on  period=1  equ=P=C  opselect=C  inp2=PCIN>>17  opr=+  inp1=P  carry=CIN  dbl_ovrd=off  block_type=constant
  Delay{1..3,20..21} (5 alike) : xbsIndex_r4/Delay  rst=off  infoeditControl=Selection of Reset will increase slice count due to use of real FFs and instead of SRLs  en=off  latency=4  dbl_ovrd=off  reg_retiming=on  block_type=delay
      settings: xl_area=[0, 0, 0, 0, 0, 0, 0]
  Delay23 : xbsIndex_r4/Delay  rst=off  infoeditControl=Selection of Reset will increase slice count due to use of real FFs and instead of SRLs  en=off  latency=3  dbl_ovrd=off  reg_retiming=on  block_type=delay
      settings: xl_area=[0, 0, 0, 0, 0, 0, 0]
  Delay24 : xbsIndex_r4/Delay  rst=off  infoeditControl=Selection of Reset will increase slice count due to use of real FFs and instead of SRLs  en=off  latency=3  dbl_ovrd=off  reg_retiming=on  block_type=delay
      settings: xl_area=[0, 0, 0, 0, 0, 0, 0]
  Delay25 : xbsIndex_r4/Delay  rst=off  infoeditControl=Selection of Reset will increase slice count due to use of real FFs and instead of SRLs  en=off  latency=3  dbl_ovrd=off  reg_retiming=on  block_type=delay
      settings: xl_area=[0, 0, 0, 0, 0, 0, 0]
  Dual Port RAM : xbsIndex_r4/Dual Port RAM  depth=2^buf_bits  initVector=1  distributed_mem=Block RAM  init_a=0  init_b=0  rst_a=off  rst_b=off  en_a=off  en_b=off  latency=4  write_mode_A=Read Before Write  write_mode_B=Read Before Write  dbl_ovrd=off  optimize=Speed  block_type=dpram
      settings: xl_area=[0, 0, 0, 0, 0, 0, 0]  block_version=10.1.3
  Terminator1 : Terminator
  deflagger : Subsystem
  input_control : Subsystem
  output_control : Subsystem
  data_out : Outport
  flag_out : Outport  Port=2
  valid_out : Outport  Port=3
  rcvd : Outport  Port=4
  time_out : Outport  Port=5
  rd_window : Outport  Port=6
  pkt_pos : Outport  Port=7
  src_out : Outport  Port=8
  wires:
  Delay1/1 -> time_out/1
  output_control/4(rd_timestamp) -> Delay1/1
  Delay25/1 -> Dual Port RAM/6
  Delay23/1 -> Dual Port RAM/5
  Delay24/1 -> Dual Port RAM/4
  input_control/1(maxcnt) -> output_control/1(maxcnt)
  input_control/3(wr_data) -> Delay23/1
  output_control/3(current_rd_window) -> Delay20/1
  Dual Port RAM/2 -> Terminator1/1
  Delay20/1 -> rd_window/1
  Delay21/1 -> valid_out/1
  Dual Port RAM/1 -> deflagger/1(din)
  Constant/1 -> Dual Port RAM/2
  output_control/2(rd_addr) -> Dual Port RAM/1
  output_control/1(rd_en) -> Delay21/1, Dual Port RAM/3
  input_control/2(wr_addr) -> Delay24/1
  input_control/4(we) -> Delay25/1
  din/1 -> input_control/1(data_in)
  valid_in/1 -> input_control/3(valid)
  eof/1 -> input_control/4(eof)
  time_in/1 -> input_control/5(time)
  src_in/1 -> input_control/6(src)
  n_brds/1 -> output_control/3(n_brds), input_control/8(n_brds)
  pkt_size/1 -> output_control/2(pkt_size), input_control/7(pkt_size)
  deflagger/2(flag) -> flag_out/1
  deflagger/3(rcvd) -> rcvd/1
  deflagger/1(dout) -> data_out/1
  flags_in/1 -> input_control/2(flag_in)
  Delay2/1 -> pkt_pos/1
  output_control/5(pkt_pos) -> Delay2/1
  Delay3/1 -> src_out/1
  output_control/6(src_out) -> Delay3/1

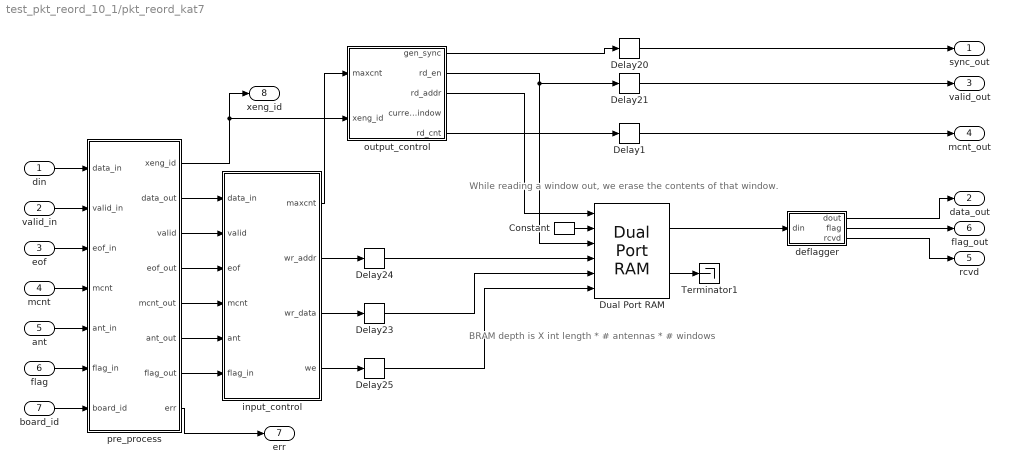
== system test_pkt_reord_10_1/pkt_reord_kat7 ==
  note: While reading a window out,
      | we erase the contents of that window.
  note: BRAM depth is
      | X int length * # antennas * # windows
  din : Inport
  valid_in : Inport  Port=2
  eof : Inport  Port=3
  mcnt : Inport  Port=4
  ant : Inport  Port=5
  flag : Inport  Port=6
  board_id : Inport  Port=7
  Constant : xbsIndex_r4/Constant  arith_type=Unsigned  const=0  n_bits=18  bin_pt=0  explicit_period=on  period=1  equ=P=C  opselect=C  inp2=PCIN>>17  opr=+  inp1=P  carry=CIN  dbl_ovrd=off  block_type=constant
  Delay1 : xbsIndex_r4/Delay  en=off  latency=3  dbl_ovrd=off  reg_retiming=on  block_type=delay
      settings: xl_area=[0, 0, 0, 0, 0, 0, 0]
  Delay20 : xbsIndex_r4/Delay  en=off  latency=3  dbl_ovrd=off  reg_retiming=on  block_type=delay
      settings: xl_area=[0, 0, 0, 0, 0, 0, 0]
  Delay21 : xbsIndex_r4/Delay  en=off  latency=3  dbl_ovrd=off  reg_retiming=on  block_type=delay
      settings: xl_area=[0, 0, 0, 0, 0, 0, 0]
  Delay23 : xbsIndex_r4/Delay  en=off  latency=2  dbl_ovrd=off  reg_retiming=on  block_type=delay
      settings: xl_area=[0, 0, 0, 0, 0, 0, 0]
  Delay24 : xbsIndex_r4/Delay  en=off  latency=2  dbl_ovrd=off  reg_retiming=on  block_type=delay
      settings: xl_area=[0, 0, 0, 0, 0, 0, 0]
  Delay25 : xbsIndex_r4/Delay  en=off  latency=2  dbl_ovrd=off  reg_retiming=on  block_type=delay
      settings: xl_area=[0, 0, 0, 0, 0, 0, 0]
  Dual Port RAM : xbsIndex_r4/Dual Port RAM  depth=2^x_int_bits * 2^ant_bits * 2^window_bits  initVector=1  distributed_mem=Block RAM  init_a=0  init_b=0  rst_a=off  rst_b=off  en_a=off  en_b=off  latency=3  write_mode_A=Read Before Write  write_mode_B=Read Before Write  dbl_ovrd=off  optimize=Area  use_rpm=off  block_type=dpram
      settings: xl_area=[0, 0, 0, 0, 0, 0, 0]  block_version=10.1.3
  Terminator1 : Terminator
  deflagger : Subsystem
  input_control : Subsystem
  output_control : Subsystem
  pre_process : Subsystem
  sync_out : Outport
  data_out : Outport  Port=2
  valid_out : Outport  Port=3
  mcnt_out : Outport  Port=4
  rcvd : Outport  Port=5
  flag_out : Outport  Port=6
  err : Outport  Port=7
  xeng_id : Outport  Port=8
  wires:
  Delay1/1 -> mcnt_out/1
  output_control/5(rd_cnt) -> Delay1/1
  Delay25/1 -> Dual Port RAM/6
  Delay23/1 -> Dual Port RAM/5
  Delay24/1 -> Dual Port RAM/4
  input_control/1(maxcnt) -> output_control/1(maxcnt)
  input_control/3(wr_data) -> Delay23/1
  output_control/1(gen_sync) -> Delay20/1
  Dual Port RAM/1 -> deflagger/1(din)
  Dual Port RAM/2 -> Terminator1/1
  Delay20/1 -> sync_out/1
  Delay21/1 -> valid_out/1
  deflagger/1(dout) -> data_out/1
  deflagger/2(flag) -> flag_out/1
  deflagger/3(rcvd) -> rcvd/1
  Constant/1 -> Dual Port RAM/2
  output_control/3(rd_addr) -> Dual Port RAM/1
  output_control/2(rd_en) -> Delay21/1, Dual Port RAM/3
  input_control/2(wr_addr) -> Delay24/1
  input_control/4(we) -> Delay25/1
  board_id/1 -> pre_process/7(board_id)
  valid_in/1 -> pre_process/2(valid_in)
  mcnt/1 -> pre_process/4(mcnt)
  din/1 -> pre_process/1(data_in)
  eof/1 -> pre_process/3(eof_in)
  ant/1 -> pre_process/5(ant_in)
  flag/1 -> pre_process/6(flag_in)
  pre_process/1(xeng_id) -> output_control/2(xeng_id), xeng_id/1
  pre_process/2(data_out) -> input_control/1(data_in)
  pre_process/3(valid) -> input_control/2(valid)
  pre_process/4(eof_out) -> input_control/3(eof)
  pre_process/5(mcnt_out) -> input_control/4(mcnt)
  pre_process/6(ant_out) -> input_control/5(ant)
  pre_process/7(flag_out) -> input_control/6(flag_in)
  pre_process/8(err) -> err/1
